simulink model "FOC_Model1"  (R2020a)
settings: Solver=FixedStepAuto  StartTime=0.0  StopTime=10.0  FixedStep=PWM_Ts  RelTol=1e-3
values from neighbouring files (symbols this model uses):
  Ki_id = Rs * Wc    (= 450)    [Motor_Parameters.m]
  Ki_iq = Rs * Wc    (= 450)    [Motor_Parameters.m]
  Ki_speed = 0.082    [Motor_Parameters.m]
  Kp_id = Ls * Wc    (= 0.42)    [Motor_Parameters.m]
  Kp_iq = Ls * Wc    (= 0.42)    [Motor_Parameters.m]
  Kp_speed = 0.8    [Motor_Parameters.m]
  PWM_Ts = 1/10000    (= 0.0001)    [Motor_Parameters.m]
undefined symbols (not defined in the file or in its folder): DiscIntNeverNeededParam
libraries: simulink x2
settings Model: Creator=HP  LastModifiedBy=HP

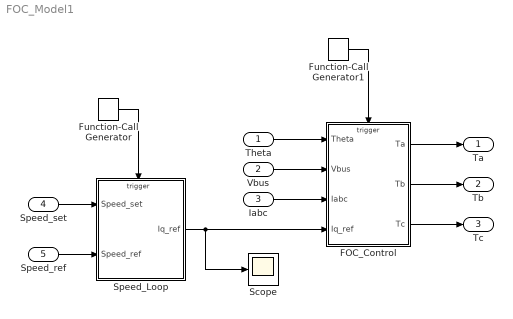
== system FOC_Model1 ==
  Theta : Inport
  Vbus : Inport  Port=2
  Iabc : Inport  Port=3  OutDataTypeStr=single
  Speed_set : Inport  Port=4  OutDataTypeStr=single
  Speed_ref : Inport  Port=5  OutDataTypeStr=single
  FOC_Control : Subsystem
  Function-Call Generator : simulink/Ports & Subsystems/Function-Call Generator  sample_time=0.001  numberOfIterations=1
  Function-Call Generator1 : simulink/Ports & Subsystems/Function-Call Generator  sample_time=0.0001  numberOfIterations=1
  Scope : Scope
  Speed_Loop : Subsystem
  Ta : Outport  OutDataTypeStr=single
  Tb : Outport  Port=2  OutDataTypeStr=single
  Tc : Outport  Port=3  OutDataTypeStr=single
  wires:
  FOC_Control/1(Ta) -> Ta/1
  FOC_Control/2(Tb) -> Tb/1
  FOC_Control/3(Tc) -> Tc/1
  Theta/1 -> FOC_Control/1(Theta)
  Vbus/1 -> FOC_Control/2(Vbus)
  Speed_set/1 -> Speed_Loop/1(Speed_set)
  Function-Call Generator/1 -> Speed_Loop/Trigger
  Function-Call Generator1/1 -> FOC_Control/Trigger
  Iabc/1 -> FOC_Control/3(Iabc)
  Speed_ref/1 -> Speed_Loop/2(Speed_ref)
  Speed_Loop/1(Iq_ref) -> Scope/1, FOC_Control/4(Iq_ref)

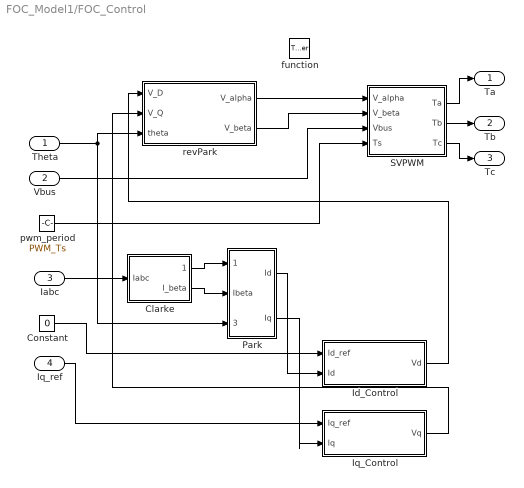
== system FOC_Model1/FOC_Control ==
  Theta : Inport  OutDataTypeStr=single
  Vbus : Inport  Port=2  OutDataTypeStr=single
  Iabc : Inport  Port=3  OutDataTypeStr=single
  Iq_ref : Inport  Port=4  OutDataTypeStr=single
  function : TriggerPort  TriggerType=function-call  VariantControl=Variant
  Clarke : Subsystem
  Constant : Constant  Value=0  OutDataTypeStr=single
  Id_Control : Subsystem
  Iq_Control : Subsystem
  Park : Subsystem
  SVPWM : Subsystem
  pwm_period : Constant  Value=PWM_Ts  OutDataTypeStr=single
  revPark : Subsystem
  Ta : Outport  OutDataTypeStr=single
  Tb : Outport  Port=2  OutDataTypeStr=single
  Tc : Outport  Port=3  OutDataTypeStr=single
  wires:
  Vbus/1 -> SVPWM/3(Vbus)
  Theta/1 -> revPark/3(theta), Park/3(Theta)
  SVPWM/1(Ta) -> Ta/1
  revPark/2(V_beta) -> SVPWM/2(V_beta)
  pwm_period/1 -> SVPWM/4(Ts)
  SVPWM/3(Tc) -> Tc/1
  SVPWM/2(Tb) -> Tb/1
  revPark/1(V_alpha) -> SVPWM/1(V_alpha)
  Iabc/1 -> Clarke/1(Iabc)
  Clarke/1(I_alpha) -> Park/1(Ialpha)
  Clarke/2(I_beta) -> Park/2(Ibeta)
  Park/1(Id) -> Id_Control/2(Id)
  Park/2(Iq) -> Iq_Control/2(Iq)
  Iq_ref/1 -> Iq_Control/1(Iq_ref)
  Id_Control/1(Vd) -> revPark/1(V_D)
  Iq_Control/1(Vq) -> revPark/2(V_Q)
  Constant/1 -> Id_Control/1(Id_ref)

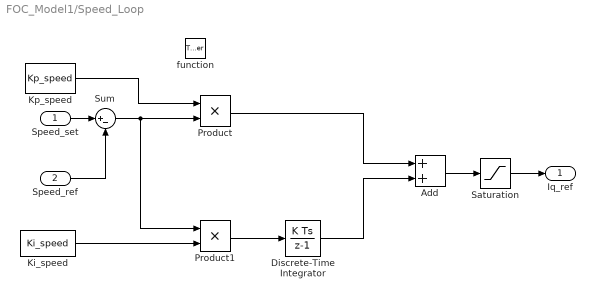
== system FOC_Model1/Speed_Loop ==
  Speed_set : Inport  OutDataTypeStr=single
  Speed_ref : Inport  Port=2  OutDataTypeStr=single
  function : TriggerPort  TriggerType=function-call  VariantControl=Variant
  Add : Sum
  Discrete-Time Integrator : DiscreteIntegrator  SampleTime=-1  ICPrevOutput=DiscIntNeverNeededParam  ICPrevScaledInput=DiscIntNeverNeededParam
  Ki_speed : Constant  Value=Ki_speed  OutDataTypeStr=single
  Kp_speed : Constant  Value=Kp_speed  OutDataTypeStr=single
  Product : Product  OutDataTypeStr=single
  Product1 : Product  OutDataTypeStr=single
  Saturation : Saturate  UpperLimit=10  LowerLimit=-10  OutDataTypeStr=single
  Sum : Sum  Inputs=|+-
  Iq_ref : Outport  OutDataTypeStr=single
  wires:
  Discrete-Time Integrator/1 -> Add/2
  Product1/1 -> Discrete-Time Integrator/1
  Add/1 -> Saturation/1
  Product/1 -> Add/1
  Speed_set/1 -> Sum/1
  Speed_ref/1 -> Sum/2
  Kp_speed/1 -> Product/1
  Sum/1 -> Product1/1, Product/2
  Saturation/1 -> Iq_ref/1
  Ki_speed/1 -> Product1/2

== system FOC_Model1/FOC_Control/Clarke ==
  note: Clarke
  Iabc : Inport  OutDataTypeStr=single
  Demux : Demux  Outputs=3
  Mux : Mux  Inputs=3
  alpha : Fcn  Expr=(u(1)-0.5*(u(2)+u(3)))*2/3
  beta : Fcn  Expr=sqrt(3)/2*(u(2)-u(3))*2/3
  I_alpha : Outport  OutDataTypeStr=single
  I_beta : Outport  Port=2  OutDataTypeStr=single
  wires:
  Iabc/1 -> Demux/1
  beta/1 -> I_beta/1
  Mux/1 -> beta/1, alpha/1
  Demux/1 -> Mux/1
  alpha/1 -> I_alpha/1
  Demux/2 -> Mux/2
  Demux/3 -> Mux/3

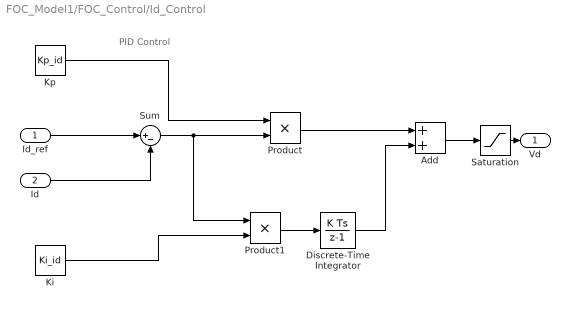
== system FOC_Model1/FOC_Control/Id_Control ==
  note: PID Control
  Id_ref : Inport  OutDataTypeStr=single
  Id : Inport  Port=2  OutDataTypeStr=single
  Add : Sum
  Discrete-Time Integrator : DiscreteIntegrator  SampleTime=-1  ICPrevOutput=DiscIntNeverNeededParam  ICPrevScaledInput=DiscIntNeverNeededParam
  Ki : Constant  Value=Ki_id  OutDataTypeStr=single
  Kp : Constant  Value=Kp_id  OutDataTypeStr=single
  Product : Product  OutDataTypeStr=single
  Product1 : Product  OutDataTypeStr=single
  Saturation : Saturate  UpperLimit=24/(sqrt(3))  LowerLimit=-24/(sqrt(3))  OutDataTypeStr=single
  Sum : Sum  Inputs=|+-
  Vd : Outport
  wires:
  Id_ref/1 -> Sum/1
  Id/1 -> Sum/2
  Sum/1 -> Product1/1, Product/2
  Kp/1 -> Product/1
  Ki/1 -> Product1/2
  Product1/1 -> Discrete-Time Integrator/1
  Product/1 -> Add/1
  Discrete-Time Integrator/1 -> Add/2
  Add/1 -> Saturation/1
  Saturation/1 -> Vd/1

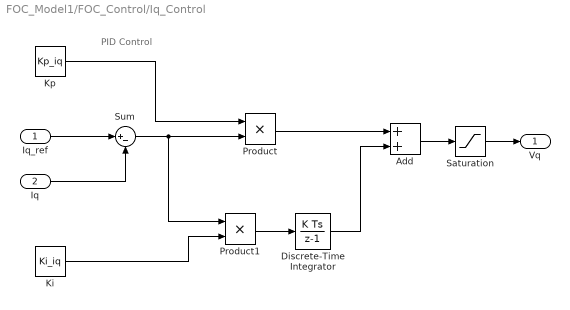
== system FOC_Model1/FOC_Control/Iq_Control ==
  note: PID Control
  Iq_ref : Inport
  Iq : Inport  Port=2
  Add : Sum
  Discrete-Time Integrator : DiscreteIntegrator  SampleTime=-1  ICPrevOutput=DiscIntNeverNeededParam  ICPrevScaledInput=DiscIntNeverNeededParam
  Ki : Constant  Value=Ki_iq  OutDataTypeStr=single
  Kp : Constant  Value=Kp_iq  OutDataTypeStr=single
  Product : Product
  Product1 : Product
  Saturation : Saturate  UpperLimit=24/(sqrt(3))  LowerLimit=-24/(sqrt(3))
  Sum : Sum  Inputs=|+-
  Vq : Outport
  wires:
  Discrete-Time Integrator/1 -> Add/2
  Product1/1 -> Discrete-Time Integrator/1
  Kp/1 -> Product/1
  Add/1 -> Saturation/1
  Ki/1 -> Product1/2
  Product/1 -> Add/1
  Sum/1 -> Product1/1, Product/2
  Iq/1 -> Sum/2
  Saturation/1 -> Vq/1
  Iq_ref/1 -> Sum/1

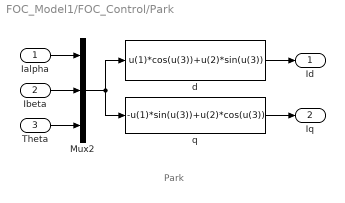
== system FOC_Model1/FOC_Control/Park ==
  note: Park
  Ialpha : Inport  OutDataTypeStr=single
  Ibeta : Inport  Port=2  OutDataTypeStr=single
  Theta : Inport  Port=3  OutDataTypeStr=single
  Mux2 : Mux  Inputs=3
  d : Fcn  Expr=u(1)*cos(u(3))+u(2)*sin(u(3))
  q : Fcn  Expr=-u(1)*sin(u(3))+u(2)*cos(u(3))
  Id : Outport  OutDataTypeStr=single
  Iq : Outport  Port=2  OutDataTypeStr=single
  wires:
  Mux2/1 -> q/1, d/1
  Ialpha/1 -> Mux2/1
  Ibeta/1 -> Mux2/2
  Theta/1 -> Mux2/3
  d/1 -> Id/1
  q/1 -> Iq/1

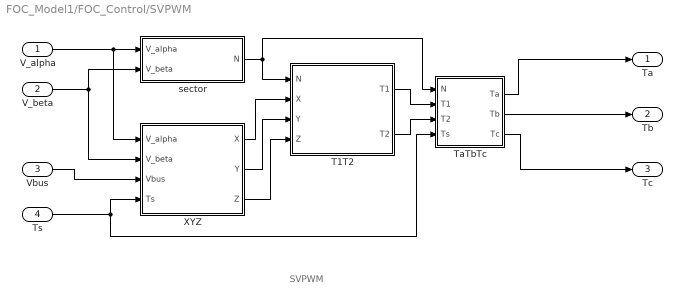
== system FOC_Model1/FOC_Control/SVPWM ==
  note: SVPWM
  V_alpha : Inport  OutDataTypeStr=single
  V_beta : Inport  Port=2  OutDataTypeStr=single
  Vbus : Inport  Port=3  OutDataTypeStr=single
  Ts : Inport  Port=4  OutDataTypeStr=single
  T1T2 : Subsystem
  TaTbTc : Subsystem
  XYZ : Subsystem
  sector : Subsystem
  Ta : Outport  OutDataTypeStr=single
  Tb : Outport  Port=2  OutDataTypeStr=single
  Tc : Outport  Port=3  OutDataTypeStr=single
  wires:
  V_alpha/1 -> sector/1(V_alpha), XYZ/1(V_alpha)
  V_beta/1 -> XYZ/2(V_beta), sector/2(V_beta)
  Ts/1 -> TaTbTc/4(Ts), XYZ/4(Ts)
  Vbus/1 -> XYZ/3(Vbus)
  sector/1(N) -> TaTbTc/1(N), T1T2/1(N)
  XYZ/1(X) -> T1T2/2(X)
  XYZ/2(Y) -> T1T2/3(Y)
  XYZ/3(Z) -> T1T2/4(Z)
  T1T2/1(T1) -> TaTbTc/2(T1)
  T1T2/2(T2) -> TaTbTc/3(T2)
  TaTbTc/1(Ta) -> Ta/1
  TaTbTc/2(Tb) -> Tb/1
  TaTbTc/3(Tc) -> Tc/1

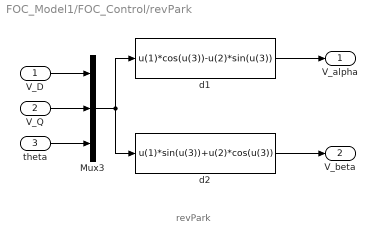
== system FOC_Model1/FOC_Control/revPark ==
  note: revPark
  V_D : Inport  OutDataTypeStr=single
  V_Q : Inport  Port=2  OutDataTypeStr=single
  theta : Inport  Port=3  OutDataTypeStr=single
  Mux3 : Mux  Inputs=3
  d1 : Fcn  Expr=u(1)*cos(u(3))-u(2)*sin(u(3))
  d2 : Fcn  Expr=u(1)*sin(u(3))+u(2)*cos(u(3))
  V_alpha : Outport  OutDataTypeStr=single
  V_beta : Outport  Port=2  OutDataTypeStr=single
  wires:
  Mux3/1 -> d1/1, d2/1
  d2/1 -> V_beta/1
  V_D/1 -> Mux3/1
  V_Q/1 -> Mux3/2
  d1/1 -> V_alpha/1
  theta/1 -> Mux3/3

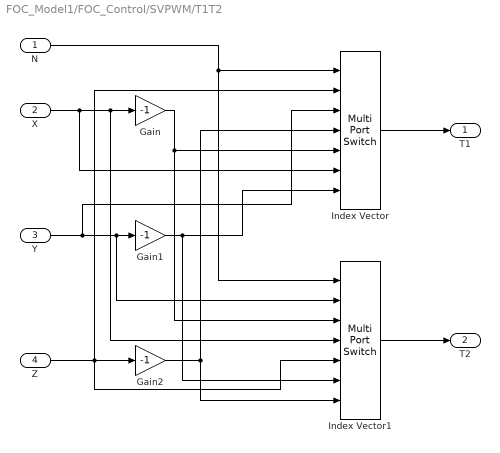
== system FOC_Model1/FOC_Control/SVPWM/T1T2 ==
  N : Inport  OutDataTypeStr=single
  X : Inport  Port=2  OutDataTypeStr=single
  Y : Inport  Port=3  OutDataTypeStr=single
  Z : Inport  Port=4  OutDataTypeStr=single
  Gain : Gain  Gain=-1
  Gain1 : Gain  Gain=-1
  Gain2 : Gain  Gain=-1
  Index Vector : MultiPortSwitch  Inputs=6
  Index Vector1 : MultiPortSwitch  Inputs=6
  T1 : Outport  OutDataTypeStr=single
  T2 : Outport  Port=2  OutDataTypeStr=single
  wires:
  X/1 -> Index Vector1/4, Gain/1, Index Vector/6
  Y/1 -> Index Vector/3, Index Vector1/2, Gain1/1
  Z/1 -> Gain2/1, Index Vector1/5, Index Vector/2
  N/1 -> Index Vector1/1, Index Vector/1
  Index Vector/1 -> T1/1
  Index Vector1/1 -> T2/1
  Gain1/1 -> Index Vector/7, Index Vector1/6
  Gain/1 -> Index Vector/5, Index Vector1/3
  Gain2/1 -> Index Vector1/7, Index Vector/4

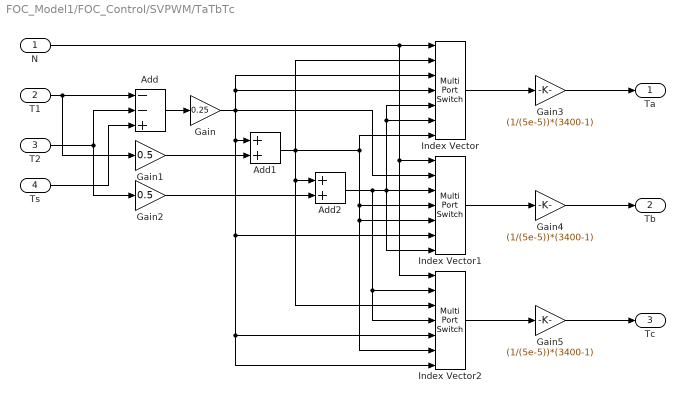
== system FOC_Model1/FOC_Control/SVPWM/TaTbTc ==
  N : Inport  OutDataTypeStr=single
  T1 : Inport  Port=2  OutDataTypeStr=single
  T2 : Inport  Port=3  OutDataTypeStr=single
  Ts : Inport  Port=4  OutDataTypeStr=single
  Add : Sum  Inputs=--+
  Add1 : Sum
  Add2 : Sum
  Gain : Gain  Gain=0.25
  Gain1 : Gain  Gain=0.5
  Gain2 : Gain  Gain=0.5
  Gain3 : Gain  Gain=(1/(5e-5))*(3400-1)
  Gain4 : Gain  Gain=(1/(5e-5))*(3400-1)
  Gain5 : Gain  Gain=(1/(5e-5))*(3400-1)
  Index Vector : MultiPortSwitch  Inputs=6
  Index Vector1 : MultiPortSwitch  Inputs=6
  Index Vector2 : MultiPortSwitch  Inputs=6
  Ta : Outport  OutDataTypeStr=single
  Tb : Outport  Port=2  OutDataTypeStr=single
  Tc : Outport  Port=3  OutDataTypeStr=single
  wires:
  T1/1 -> Add/1, Gain1/1
  T2/1 -> Gain2/1, Add/2
  Ts/1 -> Add/3
  Add/1 -> Gain/1
  Gain/1 -> Index Vector/4, Index Vector/3, Index Vector1/2, Index Vector1/6, Index Vector2/7, Index Vector2/5, Add1/1
  Gain1/1 -> Add1/2
  Gain2/1 -> Add2/2
  N/1 -> Index Vector2/1, Index Vector1/1, Index Vector/1
  Index Vector/1 -> Gain3/1
  Index Vector1/1 -> Gain4/1
  Index Vector2/1 -> Gain5/1
  Add2/1 -> Index Vector1/7, Index Vector/6, Index Vector/5, Index Vector1/3, Index Vector2/4, Index Vector2/2
  Add1/1 -> Index Vector2/3, Add2/1, Index Vector/7, Index Vector2/6, Index Vector1/5, Index Vector1/4, Index Vector/2
  Gain3/1 -> Ta/1
  Gain4/1 -> Tb/1
  Gain5/1 -> Tc/1

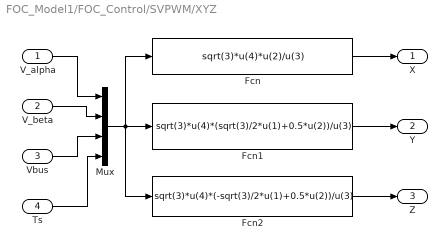
== system FOC_Model1/FOC_Control/SVPWM/XYZ ==
  V_alpha : Inport  OutDataTypeStr=single
  V_beta : Inport  Port=2  OutDataTypeStr=single
  Vbus : Inport  Port=3  OutDataTypeStr=single
  Ts : Inport  Port=4  OutDataTypeStr=single
  Fcn : Fcn  Expr=sqrt(3)*u(4)*u(2)/u(3)
  Fcn1 : Fcn  Expr=sqrt(3)*u(4)*(sqrt(3)/2*u(1)+0.5*u(2))/u(3)
  Fcn2 : Fcn  Expr=sqrt(3)*u(4)*(-sqrt(3)/2*u(1)+0.5*u(2))/u(3)
  Mux : Mux
  X : Outport  OutDataTypeStr=single
  Y : Outport  Port=2  OutDataTypeStr=single
  Z : Outport  Port=3  OutDataTypeStr=single
  wires:
  V_alpha/1 -> Mux/1
  V_beta/1 -> Mux/2
  Vbus/1 -> Mux/3
  Ts/1 -> Mux/4
  Mux/1 -> Fcn/1, Fcn1/1, Fcn2/1
  Fcn/1 -> X/1
  Fcn1/1 -> Y/1
  Fcn2/1 -> Z/1

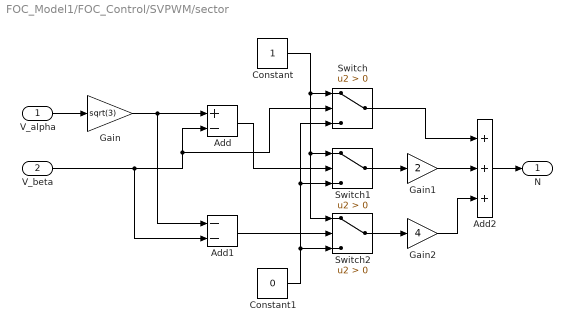
== system FOC_Model1/FOC_Control/SVPWM/sector ==
  V_alpha : Inport  OutDataTypeStr=single
  V_beta : Inport  Port=2  OutDataTypeStr=single
  Add : Sum  Inputs=+-
  Add1 : Sum  Inputs=--
  Add2 : Sum  Inputs=+++
  Constant : Constant  OutDataTypeStr=single
  Constant1 : Constant  Value=0  OutDataTypeStr=single
  Gain : Gain  Gain=sqrt(3)
  Gain1 : Gain  Gain=2
  Gain2 : Gain  Gain=4
  Switch : Switch  Criteria=u2 > Threshold
  Switch1 : Switch  Criteria=u2 > Threshold
  Switch2 : Switch  Criteria=u2 > Threshold
  N : Outport  OutDataTypeStr=single
  wires:
  V_alpha/1 -> Gain/1
  Gain/1 -> Add/1, Add1/1
  V_beta/1 -> Add1/2, Switch/2, Add/2
  Constant/1 -> Switch1/1, Switch2/1, Switch/1
  Constant1/1 -> Switch/3, Switch1/3, Switch2/3
  Add/1 -> Switch1/2
  Add1/1 -> Switch2/2
  Switch1/1 -> Gain1/1
  Switch2/1 -> Gain2/1
  Gain1/1 -> Add2/2
  Switch/1 -> Add2/1
  Gain2/1 -> Add2/3
  Add2/1 -> N/1
